simulink model "follow_path_3D"  (R2019b)
settings: Solver=FixedStepAuto  StartTime=0.0  StopTime=Inf  FixedStep=FIXED_STEP_SIZE  RelTol=1e-3
values from neighbouring files (symbols this model uses):
  GAZEBO_SYNC_DT = 0.01    [follow_path_script.m]
  POS_SUB_DT = 0.01    [follow_path_script.m]
  route = flip(route)    [Astar_3D_main.m]    (also in astar_3d.m; follow_path_script.m = astar_2d(map, start+1,end_+1); untitled.m = route + 1)
undefined symbols (not defined in the file or in its folder): Angular, Linear
libraries: robotlib x4, robotgazebolib x1, simulink x1
settings Model: SimulationMode=external  Creator=ananda  LastModifiedBy=ananda
settings OptimizationCC: EnhancedBackFolding=on  PassReuseOutputArgsAs=Individual arguments  ZeroExternalMemoryAtStartup=off  ZeroInternalMemoryAtStartup=off  MaxStackSize=64  OptimizeBlockOrder=speed  DifferentSizesBufferReuse=on  OptimizationCustomize=off  EfficientTunableParamExpr=on
settings DebuggingCC: ParameterTunabilityLossMsg=error
settings HardwareCC: ProdBitPerPointer=32  ProdBitPerSizeT=32  ProdBitPerPtrDiffT=32  ProdLargestAtomicFloat=None  ProdIntDivRoundTo=Undefined  ProdEndianess=Unspecified  ProdWordSize=32  ProdHWDeviceType=Generic->Unspecified (assume 32-bit Generic)  UseEmbeddedCoderFeatures=off
settings SFSimCC: MATLABDynamicMemAlloc=off
settings RTWCC: SystemTargetFile=ert.tlc  HardwareBoard=Robot Operating System (ROS)  TLCOptions="-aInlineSetEventsForThisBaseRateFcn=TLC_FALSE -aSuppressMultiTaskScheduler=TLC_FALSE  -aRateBasedStepFcn=0"  TemplateMakefile=ert_default_tmf  GenerateReport=on  Toolchain=Catkin  IncludeHyperlinkInReport=on  LaunchReport=on  TargetLang=C++  GenerateTraceInfo=on  GenerateTraceReport=on  GenerateTraceReportSl=on  GenerateTraceReportSf=on  GenerateTraceReportEml=on
settings CodeAppCC: ForceParamTrailComments=on  IgnoreCustomStorageClasses=off  OperatorAnnotations=on  SimulinkDataObjDesc=on  SFDataObjDesc=on  InsertBlockDesc=on
settings ERTTargetCC: SupportNonInlinedSFcns=on

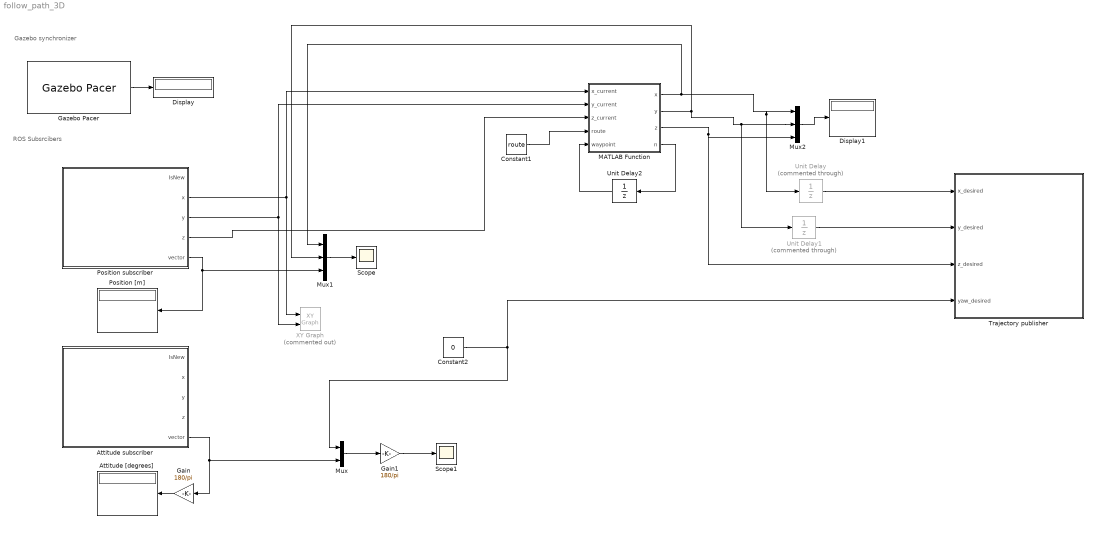
== system follow_path_3D ==
  note: Gazebo synchronizer
  note: ROS Subsrcibers
  Attitude [degrees] : Display
  Attitude subscriber : Subsystem
  Constant1 : Constant  Value=route  SampleTime=POS_SUB_DT
  Constant2 : Constant  Value=0
  Display : Display
  Display1 : Display
  Gain : Gain  Gain=180/pi
  Gain1 : Gain  Gain=180/pi
  Gazebo Pacer : robotgazebolib/Gazebo Pacer  ResetBehavior=Reset Gazebo simulation time  SampleTime=GAZEBO_SYNC_DT
      settings: SourceProductName=Robotics System Toolbox  SourceProductBaseCode=RO
  MATLAB Function : MATLAB Function  TreatAsAtomicUnit=on
  Mux : Mux  Inputs=2
  Mux1 : Mux  Inputs=3
  Mux2 : Mux  Inputs=3
  Position [m] : Display
  Position subscriber : Subsystem
  Scope : Scope
  Scope1 : Scope
  Trajectory publisher : Subsystem
  Unit Delay : UnitDelay  Commented=through  SampleTime=0.01  HasFrameUpgradeWarning=on
  Unit Delay1 : UnitDelay  Commented=through  SampleTime=0.01  HasFrameUpgradeWarning=on
  Unit Delay2 : UnitDelay  InitialCondition=1  SampleTime=POS_SUB_DT  HasFrameUpgradeWarning=on
  XY Graph : simulink/Sinks/XY Graph  Commented=on  xmin=0  xmax=10  ymin=0  ymax=10  st=0.1
  wires:
  Position subscriber/5(vector) -> Mux1/3, Position [m]/1
  Constant2/1 -> Trajectory publisher/4(yaw_desired), Mux/1
  Attitude subscriber/5(vector) -> Gain/1, Mux/2
  Gain/1 -> Attitude [degrees]/1
  Mux/1 -> Gain1/1
  Gain1/1 -> Scope1/1
  Mux1/1 -> Scope/1
  Gazebo Pacer/1 -> Display/1
  Position subscriber/2(x) -> XY Graph/1, MATLAB Function/1(x_current)
  Position subscriber/3(y) -> XY Graph/2, MATLAB Function/2(y_current)
  Mux2/1 -> Display1/1
  MATLAB Function/1(x) -> Mux1/1, Unit Delay/1, Mux2/1
  Position subscriber/4(z) -> MATLAB Function/3(z_current)
  Unit Delay/1 -> Trajectory publisher/1(x_desired)
  Unit Delay1/1 -> Trajectory publisher/2(y_desired)
  Constant1/1 -> MATLAB Function/4(route)
  Unit Delay2/1 -> MATLAB Function/5(waypoint)
  MATLAB Function/4(n) -> Unit Delay2/1
  MATLAB Function/2(y) -> Unit Delay1/1, Mux2/2, Mux1/2
  MATLAB Function/3(z) -> Mux2/3, Trajectory publisher/3(z_desired)

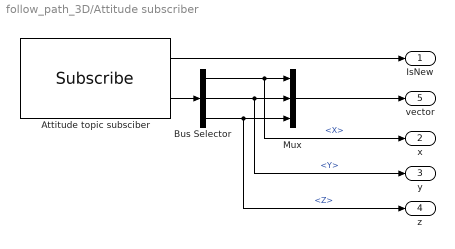
== system follow_path_3D/Attitude subscriber ==
  Attitude topic subsciber : robotlib/Subscribe  topicSource=Specify your own  topic=/ardrone/orientation_rpy  messageType=geometry_msgs/Vector3  sampleTime=ATTI_SUB_DT  messageQueueLength=1
      settings: SourceProductName=ROS Toolbox
  Bus Selector : BusSelector  OutputSignals=X,Y,Z
  Mux : Mux  Inputs=3
  IsNew : Outport
  x : Outport  Port=2
  y : Outport  Port=3
  z : Outport  Port=4
  vector : Outport  Port=5
  wires:
  Bus Selector/3 -> z/1, Mux/3  "<Z>"
  Bus Selector/2 -> y/1, Mux/2  "<Y>"
  Bus Selector/1 -> x/1, Mux/1  "<X>"
  Attitude topic subsciber/2 -> Bus Selector/1
  Attitude topic subsciber/1 -> IsNew/1
  Mux/1 -> vector/1

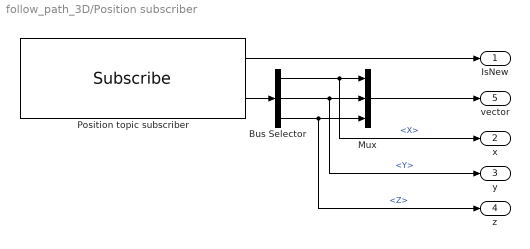
== system follow_path_3D/Position subscriber ==
  Bus Selector : BusSelector  OutputSignals=Point.X,Point.Y,Point.Z
  Mux : Mux  Inputs=3
  Position topic subscriber : robotlib/Subscribe  topicSource=Specify your own  topic=/ardrone/odometry_sensor1/position  messageType=geometry_msgs/PointStamped  sampleTime=POS_SUB_DT  messageQueueLength=1
      settings: SourceProductName=ROS Toolbox
  IsNew : Outport
  x : Outport  Port=2
  y : Outport  Port=3
  z : Outport  Port=4
  vector : Outport  Port=5
  wires:
  Bus Selector/3 -> z/1, Mux/3  "<Z>"
  Bus Selector/2 -> y/1, Mux/2  "<Y>"
  Mux/1 -> vector/1
  Bus Selector/1 -> x/1, Mux/1  "<X>"
  Position topic subscriber/2 -> Bus Selector/1
  Position topic subscriber/1 -> IsNew/1

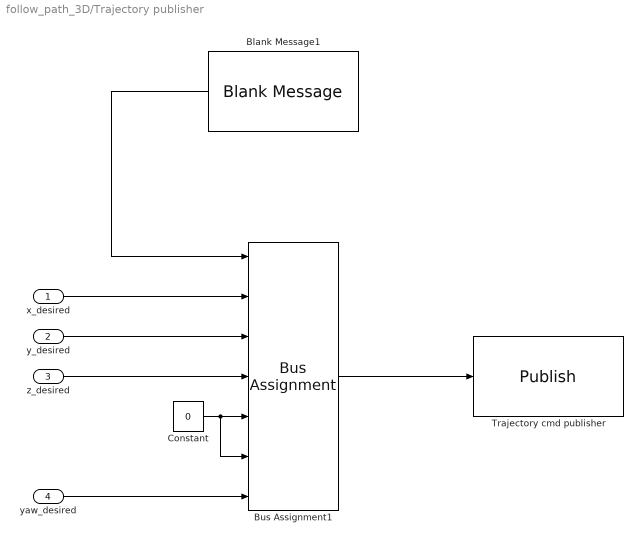
== system follow_path_3D/Trajectory publisher ==
  x_desired : Inport
  y_desired : Inport  Port=2
  z_desired : Inport  Port=3
  yaw_desired : Inport  Port=4
  Blank Message1 : robotlib/Blank Message  messageClass=Message  entityType=geometry_msgs/Twist  messageType=geometry_msgs/Twist  SampleTime=-1
      settings: SourceProductName=ROS Toolbox
  Bus Assignment1 : BusAssignment  AssignedSignals=Linear.X,Linear.Y,Linear.Z,Angular.X,Angular.Y,Angular.Z
  Constant : Constant  Value=0
  Trajectory cmd publisher : robotlib/Publish  topicSource=Specify your own  topic=/matlab/tracejtoryTwist  messageType=geometry_msgs/Twist  messageQueueLength=1
      settings: SourceProductName=ROS Toolbox
  wires:
  Blank Message1/1 -> Bus Assignment1/1
  Constant/1 -> Bus Assignment1/6, Bus Assignment1/5
  Bus Assignment1/1 -> Trajectory cmd publisher/1
  x_desired/1 -> Bus Assignment1/2
  y_desired/1 -> Bus Assignment1/3
  z_desired/1 -> Bus Assignment1/4
  yaw_desired/1 -> Bus Assignment1/7

== matlab function follow_path_3D/MATLAB Function ==
  data: x output; x_current input; y output; z output; y_current input; z_current input; route input; waypoint input; n output
function [x, y, z, n] = fcn(x_current, y_current, z_current, route, waypoint)

error = sqrt( (x_current - route(waypoint,1) + 1)^2 + (y_current - route(waypoint,2) + 1)^2 + (z_current - ((route(waypoint,3) - 1) * 2 + 1) )^2 );

if waypoint == size(route,1)
    n = waypoint
else
    if error < 0.15
        n = waypoint + 1;
    else
        n = waypoint;
    end
end

x = route(waypoint,1) - 1;
y = route(waypoint,2) - 1;
z = (route(waypoint,3) - 1) * 2 + 1;
